simulink subsystem "FCEvPerformanceCalculations"  (R2024b)
settings: Solver=VariableStepAuto  StartTime=0.0  StopTime=10.0  RelTol=1e-3
settings Model: Creator=The MathWorks, Inc.  LastModifiedBy=The MathWorks, Inc.

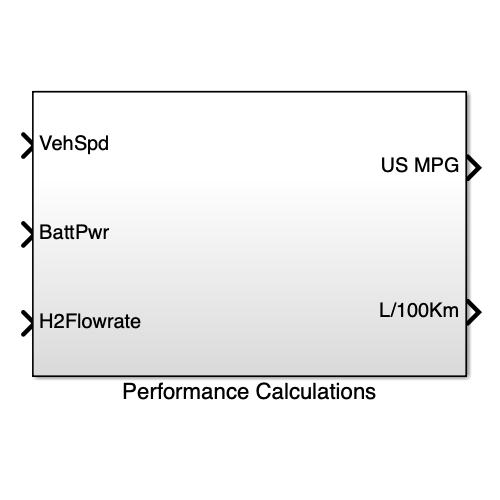
[thumbnail: Simulink's stored preview of the top-level diagram]
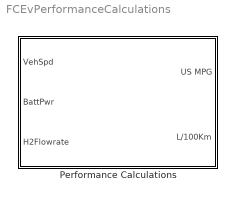
== system FCEvPerformanceCalculations ==
  Performance Calculations : Subsystem

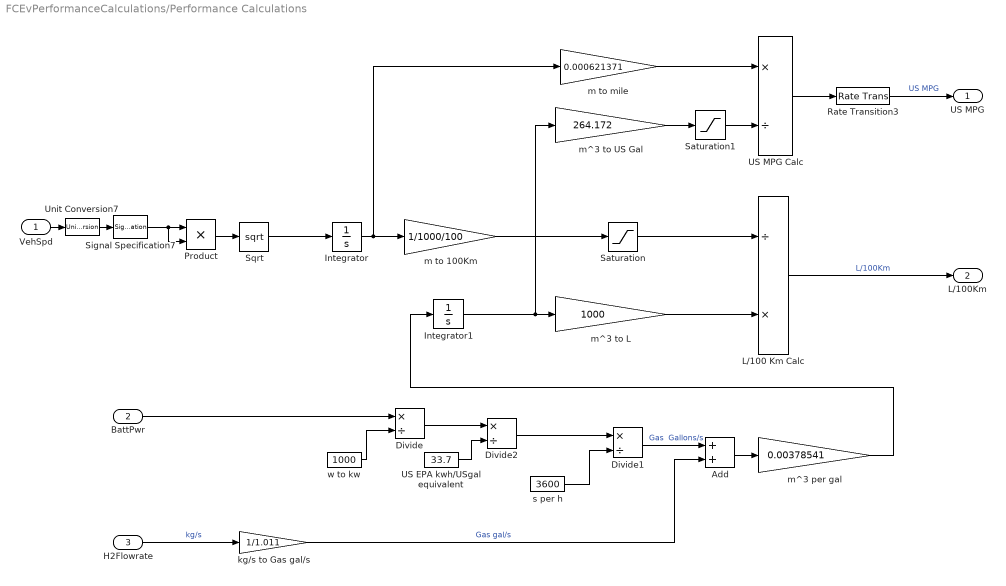
== system FCEvPerformanceCalculations/Performance Calculations ==
  VehSpd : Inport
  BattPwr : Inport  Port=2
  H2Flowrate : Inport  Port=3
  Add : Sum
  Divide : Product  Inputs=*/
  Divide1 : Product  Inputs=*/
  Divide2 : Product  Inputs=*/
  Integrator : Integrator
  Integrator1 : Integrator
  L/100 Km Calc : Product  Inputs=/*
  Product : Product
  Rate Transition3 : RateTransition  Deterministic=off
  Saturation : Saturate  UpperLimit=Inf  LowerLimit=0.001  ZeroCross=off
  Saturation1 : Saturate  UpperLimit=Inf  LowerLimit=1e-3  ZeroCross=off
  Signal Specification7 : SignalSpecification  Unit=m/s
  Sqrt : Sqrt
  US EPA kwh/USgal equivalent : Constant  Value=33.7
  US MPG Calc : Product  Inputs=*/
  Unit Conversion7 : UnitConversion
  kg/s to Gas gal/s : Gain  Gain=1/1.011
  m to 100Km : Gain  Gain=1/1000/100
  m to mile : Gain  Gain=0.000621371
  m^3 per gal : Gain  Gain=0.00378541
  m^3 to L : Gain  Gain=1000
  m^3 to US Gal : Gain  Gain=264.172
  s per h : Constant  Value=3600
  w to kw : Constant  Value=1000
  US MPG : Outport  VectorParamsAs1DForOutWhenUnconnected=off
  L/100Km : Outport  Port=2  VectorParamsAs1DForOutWhenUnconnected=off
  wires:
  Add/1 -> m^3 per gal/1
  Divide/1 -> Divide2/1
  US MPG Calc/1 -> Rate Transition3/1
  US EPA kwh/USgal equivalent/1 -> Divide2/2
  Divide2/1 -> Divide1/1
  Signal Specification7/1 -> Product/2, Product/1
  s per h/1 -> Divide1/2
  Integrator/1 -> m to mile/1, m to 100Km/1
  m^3 per gal/1 -> Integrator1/1
  m^3 to L/1 -> L/100 Km Calc/2
  Sqrt/1 -> Integrator/1
  kg/s to Gas gal/s/1 -> Add/2  "Gas gal/s"
  Unit Conversion7/1 -> Signal Specification7/1
  Product/1 -> Sqrt/1
  Saturation1/1 -> US MPG Calc/2
  H2Flowrate/1 -> kg/s to Gas gal/s/1  "kg/s"
  m to mile/1 -> US MPG Calc/1
  m^3 to US Gal/1 -> Saturation1/1
  m to 100Km/1 -> Saturation/1
  Saturation/1 -> L/100 Km Calc/1
  Integrator1/1 -> m^3 to US Gal/1, m^3 to L/1
  VehSpd/1 -> Unit Conversion7/1
  Divide1/1 -> Add/1  "Gas  Gallons/s"
  BattPwr/1 -> Divide/1
  w to kw/1 -> Divide/2
  Rate Transition3/1 -> US MPG/1  "US MPG"
  L/100 Km Calc/1 -> L/100Km/1  "L/100Km"
